simulink model "TST_StateflowLoops"  (Simulink 7.4)
settings: Solver=FixedStepDiscrete  StartTime=0.0  StopTime=10.0  FixedStep=0.02  RelTol=1e-3
settings Model: Creator=kharthforeign  LastModifiedBy=kharthforeign  BufferReuse=off
settings DataIOCC: SaveOutput=off  SignalLogging=off  SaveTime=off
settings OptimizationCC: BlockReduction=off  ConditionallyExecuteInputs=off  OptimizeBlockIOStorage=off  BufferReuse=off  ExpressionFolding=off  LocalBlockOutputs=off  InitFltsAndDblsToZero=on

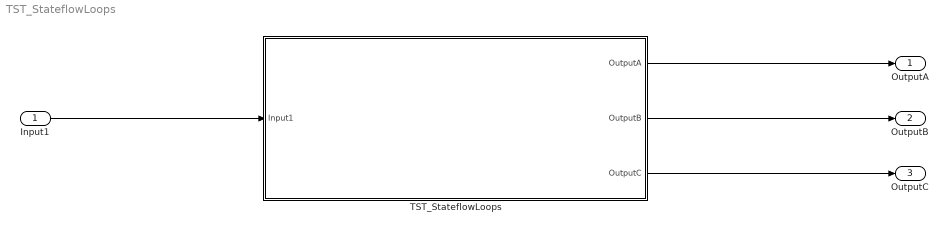
== system TST_StateflowLoops ==
  Input1 : Inport  DataType=uint32  OutDataType=fixdt(1, 16)  OutScaling=2^0  OutDataTypeStr=uint32  BusOutputAsStruct=on
  TST_StateflowLoops : Subsystem  TreatAsAtomicUnit=on
  OutputA : Outport  PortDimensions=1  DataType=double  OutDataType=fixdt(1, 16)  OutScaling=2^0  OutDataTypeStr=double
  OutputB : Outport  Port=2  PortDimensions=1  DataType=double  OutDataType=Enum: DIL_VmmGsFcsCommandsMessage_LatApModeCmd  OutDataTypeStr=double
  OutputC : Outport  Port=3  PortDimensions=1  DataType=double  OutDataType=fixdt(1, 16)  OutScaling=2^0  OutDataTypeStr=double
  wires:
  Input1/1 -> TST_StateflowLoops/1(Input1)
  TST_StateflowLoops/1(OutputA) -> OutputA/1
  TST_StateflowLoops/2(OutputB) -> OutputB/1
  TST_StateflowLoops/3(OutputC) -> OutputC/1

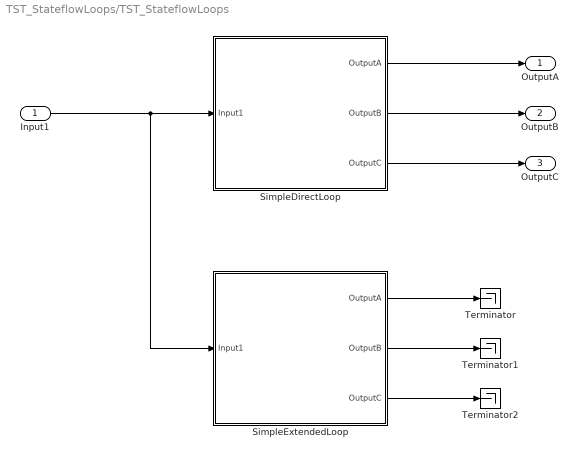
== system TST_StateflowLoops/TST_StateflowLoops ==
  Input1 : Inport  DataType=uint32  OutDataType=fixdt(1, 16)  OutScaling=2^0  OutDataTypeStr=uint32  BusOutputAsStruct=on
  SimpleDirectLoop : Stateflow chart
  SimpleExtendedLoop : Stateflow chart
  Terminator : Terminator
  Terminator1 : Terminator
  Terminator2 : Terminator
  OutputA : Outport  PortDimensions=1  DataType=double  OutDataType=fixdt(1, 16)  OutScaling=2^0  OutDataTypeStr=double
  OutputB : Outport  Port=2  PortDimensions=1  DataType=double  OutDataType=Enum: DIL_VmmGsFcsCommandsMessage_LatApModeCmd  OutDataTypeStr=double
  OutputC : Outport  Port=3  PortDimensions=1  DataType=double  OutDataType=fixdt(1, 16)  OutScaling=2^0  OutDataTypeStr=double
  wires:
  SimpleDirectLoop/1(OutputA) -> OutputA/1
  SimpleDirectLoop/2(OutputB) -> OutputB/1
  SimpleDirectLoop/3(OutputC) -> OutputC/1
  Input1/1 -> SimpleDirectLoop/1(Input1), SimpleExtendedLoop/1(Input1)
  SimpleExtendedLoop/1(OutputA) -> Terminator/1
  SimpleExtendedLoop/2(OutputB) -> Terminator1/1
  SimpleExtendedLoop/3(OutputC) -> Terminator2/1

== stateflow chart TST_StateflowLoops/SimpleDirectLoop ==
  note: simple single-transition loop
  (junction 5) -> (junction 5) [order 2] : [A]{OutputA = 1;} %loop1.1
  (junction 5) -> (junction 4) [order 3] : %safe else to A
  (default) -> (junction 5) : %default
  (junction 5) -> (junction 6) [order 1] : [B]{OutputB = 1;} %else to A
  (junction 6) -> (junction 7) [order 1] : [C]{OutputC = 1;}
  (junction 6) -> (junction 8) [order 2] : %else to C
  data: Input1 input uint32; OutputA output double =1; OutputB output double =2; OutputC output double =3; Local local uint32 =0; A local boolean; B local boolean; C local boolean

== stateflow chart TST_StateflowLoops/SimpleExtendedLoop ==
  note: loop starts at this transition
  note: simple loop consisting of several
      | transitions
  (junction 28) -> (junction 29) [order 1] : [A]{OutputA = 1;} %loop1.1
  (junction 28) -> (junction 27) [order 2] : %else to A
  (default) -> (junction 28) : %default
  (junction 29) -> (junction 30) : %loop1.2
  (junction 30) -> (junction 31) [order 1] : [B]{OutputB = 1;}%loop1.3
  (junction 31) -> (junction 28) : %loop1.4
  (junction 30) -> (junction 32) [order 2] : %else to B
  data: Input1 input uint32; OutputA output double =1; OutputB output double =2; OutputC output double =3; Local local uint32 =0; A local boolean; B local boolean; C local boolean
